simulink model "model"  (Simulink 9.0)
settings: Solver=ode3  StartTime=0.0  StopTime=inf  FixedStep=0.0001  RelTol=1e-3  EnableMultiTasking=on
libraries: slrtlib x6, xpcquanserlib x6, simulink x3
settings Model: Creator=Ninad  LastModifiedBy=Joshua  SimulationMode=external
settings SolverCC: ConcurrentTasks=on
settings DataIOCC: LimitDataPoints=on
settings OptimizationCC: BlockReduction=off  OptimizeBlockIOStorage=off  BufferReuse=off  GlobalBufferReuse=off  ExpressionFolding=off  ExpressionDepthLimit=2147483647  LocalBlockOutputs=off
settings DebuggingCC: SolverPrmCheckMsg=warning  FcnCallInpInsideContextMsg=warning  StateNameClashWarn=warning  StrictBusMsg=Warning
settings HardwareCC: ProdIntDivRoundTo=Zero  ProdEndianess=LittleEndian  ProdLongLongMode=on  ProdHWDeviceType=Generic->32-bit x86 compatible
settings RTWCC: SystemTargetFile=slrt.tlc  TemplateMakefile=slrt_default_tmf  Description=Simulink Real-Time  CodeExecutionProfiling=on  RTWCompilerOptimization=on
settings SimulinkRealTimeCC: GeneratePreprocessorConditionals=Disable all
settings ConfigComp: CovSFcnEnable=off

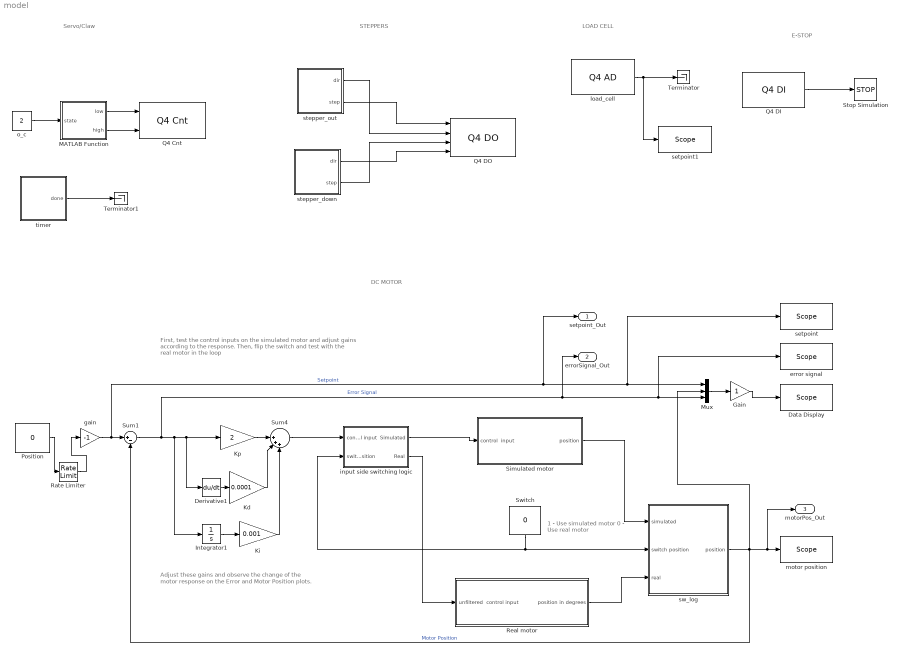
== system model ==
  note: E-STOP
  note: Adjust these gains and observe the change of the
      | motor response on the Error and Motor Position
      | plots.
  note: First, test the control inputs on the simulated motor and
      | adjust gains according to the response. Then, flip the switch and
      | test with the real motor in the loop
  note: 1 - Use simulated motor
      | 0 - Use real motor
  note: STEPPERS
  note: Servo/Claw
  note: DC MOTOR
  note: LOAD CELL
  Data Display : slrtlib/Displays and Logging/Scope   scopeno=3  scopetype=Target  autostart=on  viewmode=Numerical  formatstr="'Setpoint        %3.2f,Motor Position  %3.2f,Error Signal    %3.2f'"  grid=on  ylimits=[0,170]  nosamples=200  noprepostsamples=0  interleave=10  triggermode=FreeRun  triggersignal=1  trigsignalfromport=off  triggerlevel=0.0  triggerslope=Either  triggerscope=1  triggersample=0  filename=data.dat  mode=Lazy  writesize=512  autorestart=off  dynamicfilemode=off  maxwritefilesize=512*1024^2
  Derivative1 : Derivative
  Gain : Gain
  Integrator1 : Integrator
  Kd : Gain  Gain=0.0001
  Ki : Gain  Gain=0.001
  Kp : Gain  Gain=2
  MATLAB Function : MATLAB Function  TreatAsAtomicUnit=on
  Mux : Mux  Inputs=3
  Position : Constant  Value=0  OutDataTypeStr=double
  "Q4 Cnt " : xpcquanserlib/Counter/Q4 Cnt   channel=[1]  mode=1  showArm=[0]  reset=[1]  initLoCount=[0]  initHiCount=[0]  sampleTime=.0001  slot=-1
      settings: SourceProductName=Simulink Real-Time  SourceProductBaseCode=XP
  "Q4 DI " : xpcquanserlib/Digital Input/Q4 DI   channel=[5]  sampleTime=0.0001  slot=-1
      settings: SourceProductName=Simulink Real-Time  SourceProductBaseCode=XP
  "Q4 DO " : xpcquanserlib/Digital Output/Q4 DO   channel=[1 2 3 4]  reset=[1]  initValue=[0]  sampleTime=.0001  slot=-1
      settings: SourceProductName=Simulink Real-Time  SourceProductBaseCode=XP
  Rate Limiter : RateLimiter  RisingSlewLimit=15  FallingSlewLimit=-15  SampleTimeMode=inherited
  Real motor : Subsystem
  Simulated motor : Subsystem
  Stop Simulation : Stop
  Sum1 : Sum  Inputs=|+-
  Sum4 : Sum  Inputs=||+++
  Switch : Constant  Value=0
  Terminator : Terminator
  Terminator1 : Terminator
  error signal : slrtlib/Displays and Logging/Scope   scopeno=2  scopetype=Target  autostart=on  viewmode=Graphical rolling  formatstr='%15.6f'  grid=on  ylimits=[-180,180]  nosamples=500  noprepostsamples=0  interleave=10  triggermode=FreeRun  triggersignal=1  trigsignalfromport=off  triggerlevel=0.0  triggerslope=Either  triggerscope=1  triggersample=0  filename=data.dat  mode=Lazy  writesize=512  autorestart=off  dynamicfilemode=off  maxwritefilesize=512*1024^2
  gain : Gain  Gain=-1
  input side switching logic : Subsystem
  load_cell : xpcquanserlib/A//D/Q4 AD  channel=[1]  sampleTime=0.001  slot=-1
      settings: SourceProductName=Simulink Real-Time  SourceProductBaseCode=XP
  motor position : slrtlib/Displays and Logging/Scope   scopeno=7  scopetype=Target  autostart=on  viewmode=Graphical rolling  formatstr='%15.6f'  grid=on  ylimits=[-180,180]  nosamples=500  noprepostsamples=0  interleave=10  triggermode=FreeRun  triggersignal=1  trigsignalfromport=off  triggerlevel=0.0  triggerslope=Either  triggerscope=1  triggersample=0  filename=data.dat  mode=Lazy  writesize=512  autorestart=off  dynamicfilemode=off  maxwritefilesize=512*1024^2
  o_c : Constant  Value=2
  setpoint : slrtlib/Displays and Logging/Scope   scopeno=1  scopetype=Target  autostart=on  viewmode=Graphical rolling  formatstr='%15.6f'  grid=on  ylimits=[-180,180]  nosamples=500  noprepostsamples=0  interleave=10  triggermode=FreeRun  triggersignal=1  trigsignalfromport=off  triggerlevel=0.0  triggerslope=Either  triggerscope=1  triggersample=0  filename=data.dat  mode=Lazy  writesize=512  autorestart=off  dynamicfilemode=off  maxwritefilesize=512*1024^2
  setpoint1 : slrtlib/Displays and Logging/Scope   scopeno=4  scopetype=Target  autostart=on  viewmode=Graphical rolling  formatstr='%15.6f'  grid=on  ylimits=[-10 10]  nosamples=500  noprepostsamples=0  interleave=1  triggermode=FreeRun  triggersignal=1  trigsignalfromport=off  triggerlevel=0.0  triggerslope=Either  triggerscope=1  triggersample=0  filename=data.dat  mode=Lazy  writesize=512  autorestart=off  dynamicfilemode=off  maxwritefilesize=512*1024^2
  stepper_down : Subsystem
  stepper_out : Subsystem
  sw_log : Subsystem
  timer : Subsystem
  setpoint_Out : Outport
  errorSignal_Out : Outport  Port=2
  motorPos_Out : Outport  Port=3
  wires:
  Kp/1 -> Sum4/1
  Kd/1 -> Sum4/2
  Derivative1/1 -> Kd/1
  Integrator1/1 -> Ki/1
  Ki/1 -> Sum4/3
  gain/1 -> Sum1/1, Mux/1, setpoint/1, setpoint_Out/1  "Setpoint"
  input side switching logic/1(Simulated) -> Simulated motor/1(control  input)
  input side switching logic/2(Real) -> Real motor/1(unfiltered  control input)
  Simulated motor/1(position) -> sw_log/1(simulated)
  Real motor/1(position in degrees) -> sw_log/3(real)
  sw_log/1(position) -> Mux/2, Sum1/2, motor position/1, motorPos_Out/1  "Motor Position"
  Sum4/1 -> input side switching logic/1(control input)
  Switch/1 -> input side switching logic/2(switch  position), sw_log/2(switch position)
  Gain/1 -> Data Display/1
  Mux/1 -> Gain/1
  Sum1/1 -> Kp/1, Derivative1/1, Integrator1/1, Mux/3, error signal/1, errorSignal_Out/1  "Error Signal"
  "Q4 DI "/1 -> Stop Simulation/1
  MATLAB Function/1(low) -> "Q4 Cnt "/1
  MATLAB Function/2(high) -> "Q4 Cnt "/2
  o_c/1 -> MATLAB Function/1(state)
  load_cell/1 -> setpoint1/1, Terminator/1
  timer/1(done) -> Terminator1/1
  stepper_out/2(step) -> "Q4 DO "/1
  stepper_out/1(dir) -> "Q4 DO "/2
  stepper_down/1(dir) -> "Q4 DO "/4
  stepper_down/2(step) -> "Q4 DO "/3
  Position/1 -> Rate Limiter/1
  Rate Limiter/1 -> gain/1

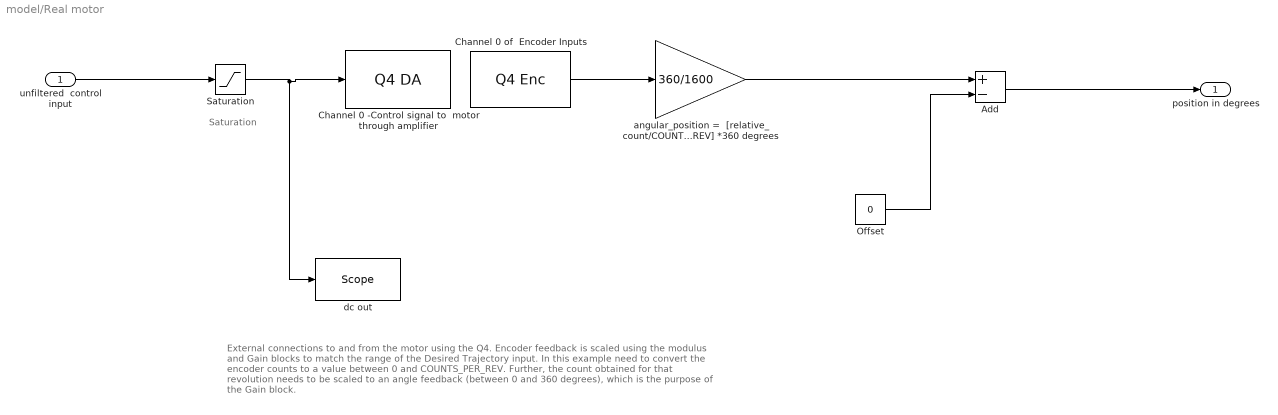
== system model/Real motor ==
  note: Saturation
  note: External connections to and from the motor using the Q4.
      |
      | Encoder feedback is scaled using the modulus and Gain blocks to
      | match the range of the Desired Trajectory input.
      |
      | In this example need to convert the encoder counts to a value between 0 and COUNTS_PER_REV.
      | Further, the count obtained for that revolution needs to be scaled to an angle feedback (between
      | 0 and 360 degrees), which is the purpose of the Gain block.
  unfiltered  control input : Inport
  Add : Sum  Inputs=+-
  "Channel 0 -Control signal to  motor through amplifier " : xpcquanserlib/D//A/Q4 DA   channel=[1]  range=[-10]  simul=off  reset=[1]  initValue=[0]  sampleTime=.0001  slot=-1
      settings: SourceProductName=Simulink Real-Time  SourceProductBaseCode=XP
  "Channel 0 of  Encoder Inputs " : xpcquanserlib/Incremental Encoder/Q4 Enc   channel=1  initialCount=[0]  prescale=[1]  quadrature=[4]  mode=[0]  synchronousIndex=[0]  indexPolarity=[0]  preserveCounts=[0]  sampleTime=.0001  slot=-1
      settings: SourceProductName=Simulink Real-Time  SourceProductBaseCode=XP
  Offset : Constant  Value=0
  Saturation : Saturate  UpperLimit=8  LowerLimit=-8
  angular_position =  [relative_count/COUNTS_PER_REV] *360 degrees : Gain  Gain=360/1600
  dc out : slrtlib/Displays and Logging/Scope   scopeno=8  scopetype=Target  autostart=on  viewmode=Graphical rolling  formatstr='%15.6f'  grid=on  ylimits=[-10, 10]  nosamples=500  noprepostsamples=0  interleave=10  triggermode=FreeRun  triggersignal=1  trigsignalfromport=off  triggerlevel=0.0  triggerslope=Either  triggerscope=1  triggersample=0  filename=data.dat  mode=Lazy  writesize=512  autorestart=off  dynamicfilemode=off  maxwritefilesize=512*1024^2
  position in degrees : Outport
  wires:
  Saturation/1 -> "Channel 0 -Control signal to  motor through amplifier "/1, dc out/1
  "Channel 0 of  Encoder Inputs "/1 -> angular_position =  [relative_count/COUNTS_PER_REV] *360 degrees/1
  unfiltered  control input/1 -> Saturation/1
  Add/1 -> position in degrees/1
  angular_position =  [relative_count/COUNTS_PER_REV] *360 degrees/1 -> Add/1
  Offset/1 -> Add/2

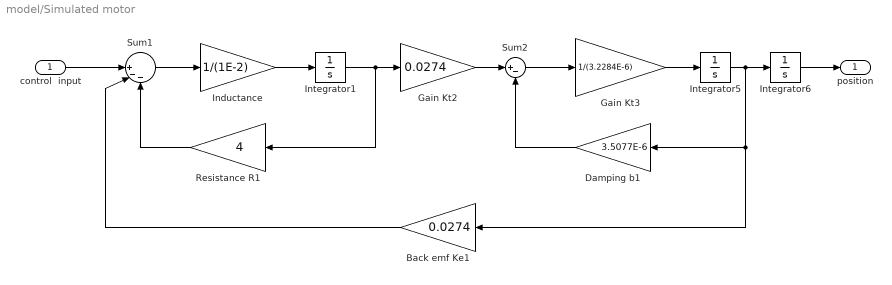
== system model/Simulated motor ==
  control  input : Inport
  Back emf Ke1 : Gain  Gain=0.0274
  Damping b1 : Gain  Gain=3.5077E-6
  Gain Kt2 : Gain  Gain=0.0274
  Gain Kt3 : Gain  Gain=1/(3.2284E-6)
  Inductance : Gain  Gain=1/(1E-2)
  Integrator1 : Integrator
  Integrator5 : Integrator
  Integrator6 : Integrator
  Resistance R1 : Gain  Gain=4
  Sum1 : Sum  Inputs=||+--
  Sum2 : Sum  Inputs=|+-
  position : Outport
  wires:
  Sum1/1 -> Inductance/1
  Inductance/1 -> Integrator1/1
  Integrator1/1 -> Gain Kt2/1, Resistance R1/1
  Gain Kt2/1 -> Sum2/1
  Sum2/1 -> Gain Kt3/1
  Gain Kt3/1 -> Integrator5/1
  Integrator5/1 -> Integrator6/1, Back emf Ke1/1, Damping b1/1
  Back emf Ke1/1 -> Sum1/2
  Damping b1/1 -> Sum2/2
  Resistance R1/1 -> Sum1/3
  Integrator6/1 -> position/1
  control  input/1 -> Sum1/1

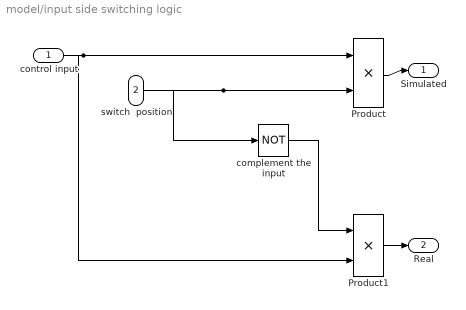
== system model/input side switching logic ==
  control input : Inport
  switch  position : Inport  Port=2
  Product : Product  RndMeth=Zero
  Product1 : Product  RndMeth=Zero
  complement the input : Logic  Operator=NOT  AllPortsSameDT=off  OutDataTypeStr=boolean
  Simulated : Outport
  Real : Outport  Port=2
  wires:
  control input/1 -> Product1/2, Product/1
  complement the input/1 -> Product1/1
  switch  position/1 -> complement the input/1, Product/2
  Product/1 -> Simulated/1
  Product1/1 -> Real/1

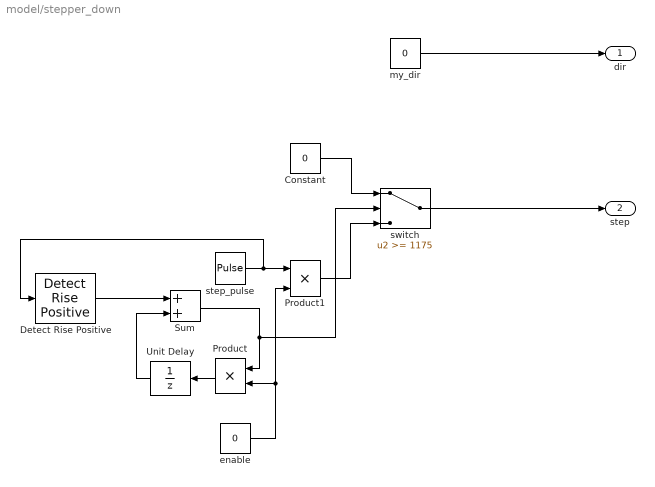
== system model/stepper_down ==
  Constant : Constant  Value=0
  Detect Rise Positive : simulink/Logic and Bit Operations/Detect Rise Positive  vinit=0  OutDataTypeStr=uint8
  Product : Product  OutDataTypeStr=uint32
  Product1 : Product  OutDataTypeStr=uint32
  Sum : Sum  OutDataTypeStr=uint32  SaturateOnIntegerOverflow=on
  Unit Delay : UnitDelay  SampleTime=-1
  enable : Constant  Value=0  OutDataTypeStr=uint32
  my_dir : Constant  Value=0
  step_pulse : DiscretePulseGenerator  PulseType=Time based  Period=0.002  PulseWidth=50
  switch : Switch  Threshold=1175
  dir : Outport
  step : Outport  Port=2
  wires:
  my_dir/1 -> dir/1
  switch/1 -> step/1
  Detect Rise Positive/1 -> Sum/1
  Sum/1 -> switch/2, Product/1
  enable/1 -> Product1/2, Product/2
  Product/1 -> Unit Delay/1
  Unit Delay/1 -> Sum/2
  step_pulse/1 -> Product1/1, Detect Rise Positive/1
  Constant/1 -> switch/1
  Product1/1 -> switch/3

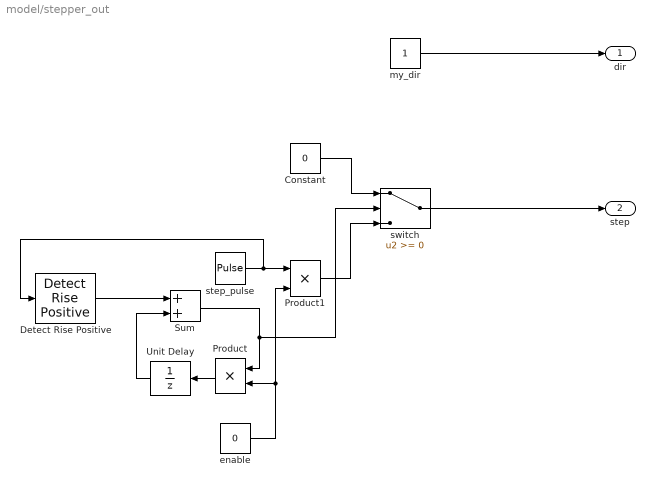
== system model/stepper_out ==
  Constant : Constant  Value=0
  Detect Rise Positive : simulink/Logic and Bit Operations/Detect Rise Positive  vinit=0  OutDataTypeStr=uint8
  Product : Product  OutDataTypeStr=uint32
  Product1 : Product  OutDataTypeStr=uint32
  Sum : Sum  OutDataTypeStr=uint32  SaturateOnIntegerOverflow=on
  Unit Delay : UnitDelay  SampleTime=-1
  enable : Constant  Value=0  OutDataTypeStr=uint32
  my_dir : Constant
  step_pulse : DiscretePulseGenerator  PulseType=Time based  Period=0.01  PulseWidth=50
  switch : Switch
  dir : Outport
  step : Outport  Port=2
  wires:
  my_dir/1 -> dir/1
  switch/1 -> step/1
  Detect Rise Positive/1 -> Sum/1
  Sum/1 -> switch/2, Product/1
  enable/1 -> Product1/2, Product/2
  Product/1 -> Unit Delay/1
  Unit Delay/1 -> Sum/2
  step_pulse/1 -> Product1/1, Detect Rise Positive/1
  Constant/1 -> switch/1
  Product1/1 -> switch/3

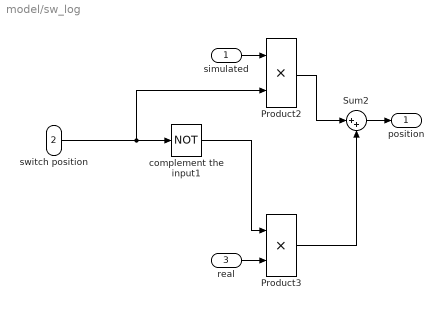
== system model/sw_log ==
  simulated : Inport
  switch position : Inport  Port=2
  real : Inport  Port=3
  Product2 : Product  RndMeth=Zero
  Product3 : Product  RndMeth=Zero
  Sum2 : Sum  Inputs=|++
  complement the input1 : Logic  Operator=NOT  AllPortsSameDT=off  OutDataTypeStr=boolean
  position : Outport
  wires:
  complement the input1/1 -> Product3/1
  Product2/1 -> Sum2/1
  Product3/1 -> Sum2/2
  switch position/1 -> Product2/2, complement the input1/1
  simulated/1 -> Product2/1
  Sum2/1 -> position/1
  real/1 -> Product3/2

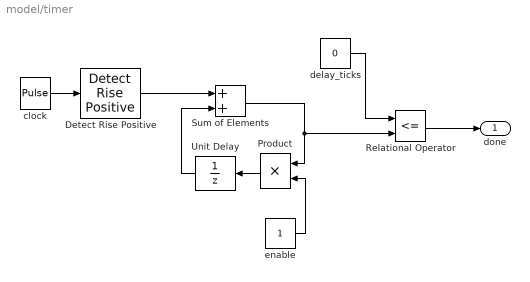
== system model/timer ==
  Detect Rise Positive : simulink/Logic and Bit Operations/Detect Rise Positive  vinit=0  OutDataTypeStr=uint8
  Product : Product
  Relational Operator : RelationalOperator  Operator=<=  OutDataTypeStr=boolean  RndMeth=Simplest
  Sum of Elements : Sum  SaturateOnIntegerOverflow=on
  Unit Delay : UnitDelay  SampleTime=-1
  clock : DiscretePulseGenerator  PulseType=Time based  Period=0.01  PulseWidth=50
  delay_ticks : Constant  Value=0
  enable : Constant
  done : Outport
  wires:
  Relational Operator/1 -> done/1
  Detect Rise Positive/1 -> Sum of Elements/1
  Sum of Elements/1 -> Product/1, Relational Operator/2
  enable/1 -> Product/2
  Product/1 -> Unit Delay/1
  Unit Delay/1 -> Sum of Elements/2
  clock/1 -> Detect Rise Positive/1
  delay_ticks/1 -> Relational Operator/1

== matlab function MATLAB Function ==
  data: state input double; low output double; high output double
function [low,high] = fcn(state)

period = 20e-3;

step = 30e-9;

if state == 1
    time_high = 0.73e-3;
elseif state == 2
    time_high = 0.65e-3;
else
    time_high = 0.9e-3;
end

low = round((period-time_high)/step);
high = round(time_high/step);


end
